simulink model "ISOtoIO"  (R2017a)
settings: Solver=VariableStepAuto  StartTime=0.0  StopTime=10.0  MaxStep=0.01  RelTol=1e-3
settings Model: Creator=drone  LastModifiedBy=drone

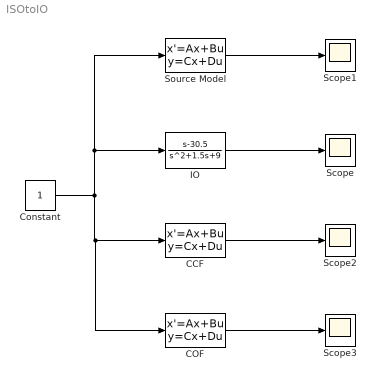
== system ISOtoIO ==
  CCF : StateSpace  A=[0 1; -9 -1.5]  B=[0; 1]  C=[-30.5 1]  D=0  X0=0
  COF : StateSpace  A=[0 -9; 1 -1.5]  B=[-30.5; 1]  C=[0 1]  D=0  X0=0
  Constant : Constant
  IO : TransferFcn  Numerator=[1 -30.5]  Denominator=[1 1.5 9]
  Scope{,1..3} (4 alike) : Scope
  Source Model : StateSpace  A=[0.5 -10; 1 -2]  B=[0; 1]  C=[3 1]  D=0  X0=0
  wires:
  CCF/1 -> Scope2/1
  Source Model/1 -> Scope1/1
  IO/1 -> Scope/1
  Constant/1 -> Source Model/1, IO/1, COF/1, CCF/1
  COF/1 -> Scope3/1
